simulink model "BLDC_Model"  (R2020a)
settings: Solver=VariableStepAuto  StartTime=0.0  StopTime=10.0  RelTol=1e-3
settings Model: Creator=DELL  LastModifiedBy=DELL

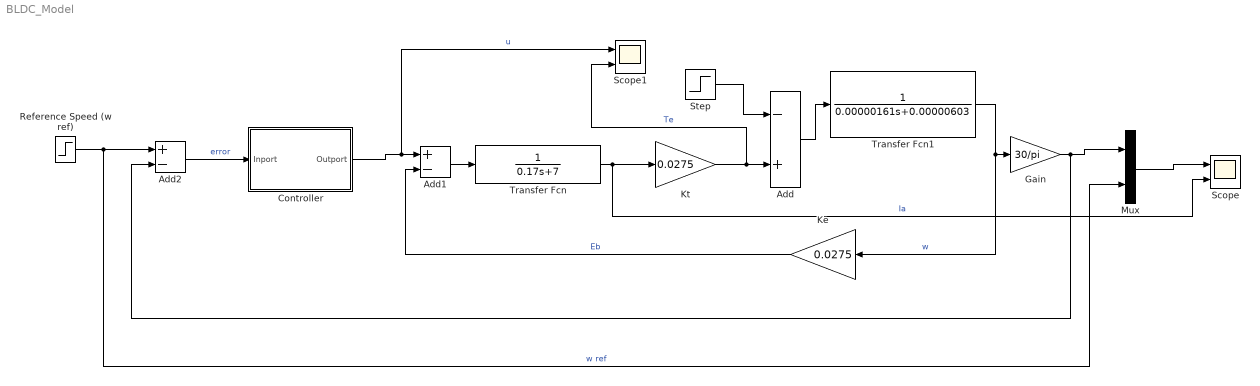
== system BLDC_Model ==
  Add : Sum  Inputs=-+
  Add1 : Sum  Inputs=+-
  Add2 : Sum  Inputs=+-
  Controller : Subsystem
  Gain : Gain  Gain=30/pi
  Ke : Gain  Gain=0.0275
  Kt : Gain  Gain=0.0275
  Mux : Mux  Inputs=2
  Reference Speed (w ref) : Step  SampleTime=0
  Scope : Scope  NumInputPorts=2
  Scope1 : Scope  NumInputPorts=2
  Step : Step  Time=0.1  After=10  SampleTime=0
  Transfer Fcn : TransferFcn  Denominator=[0.17 7]
  Transfer Fcn1 : TransferFcn  Denominator=[0.00000161 0.00000603]
  wires:
  Add1/1 -> Transfer Fcn/1
  Transfer Fcn/1 -> Scope/2, Kt/1  "Ia"
  Kt/1 -> Scope1/2, Add/2  "Te"
  Step/1 -> Add/1
  Add/1 -> Transfer Fcn1/1
  Mux/1 -> Scope/1
  Reference Speed (w ref)/1 -> Mux/2, Add2/1  "w ref"
  Add2/1 -> Controller/1(Inport)  "error"
  Transfer Fcn1/1 -> Ke/1, Gain/1  "w"
  Ke/1 -> Add1/2  "Eb"
  Controller/1(Outport) -> Scope1/1, Add1/1  "u"
  Gain/1 -> Mux/1, Add2/2

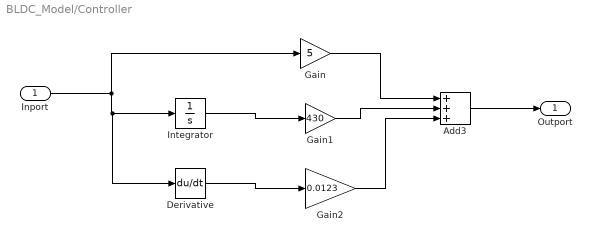
== system BLDC_Model/Controller ==
  Inport : Inport
  Add3 : Sum  Inputs=+++
  Derivative : Derivative
  Gain : Gain  Gain=5
  Gain1 : Gain  Gain=430
  Gain2 : Gain  Gain=0.0123
  Integrator : Integrator
  Outport : Outport
  wires:
  Derivative/1 -> Gain2/1
  Gain1/1 -> Add3/2
  Inport/1 -> Gain/1, Derivative/1, Integrator/1
  Integrator/1 -> Gain1/1
  Gain/1 -> Add3/1
  Add3/1 -> Outport/1
  Gain2/1 -> Add3/3
